simulink model "MyobsvIntegralSimul"  (R2021b)
settings: Solver=VariableStepAuto  StartTime=0.0  StopTime=200  RelTol=1e-3
undefined symbols (not defined in the file): A, B, C, F, G, Kd, Ki, L, Ts, x0, x_esht_0
settings Model: Creator=tanzc  LastModifiedBy=tanzc
settings DataIOCC: ReturnWorkspaceOutputs=off

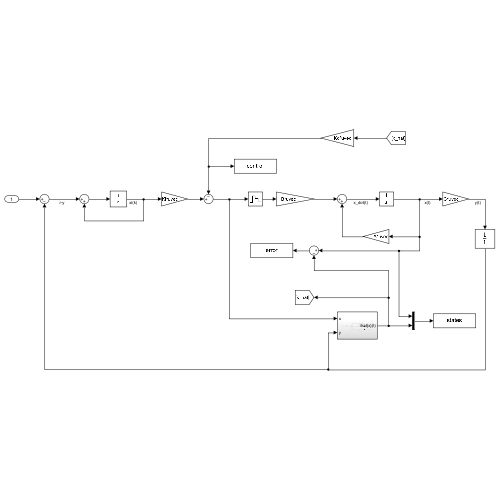
[thumbnail: Simulink's stored preview of the top-level diagram]
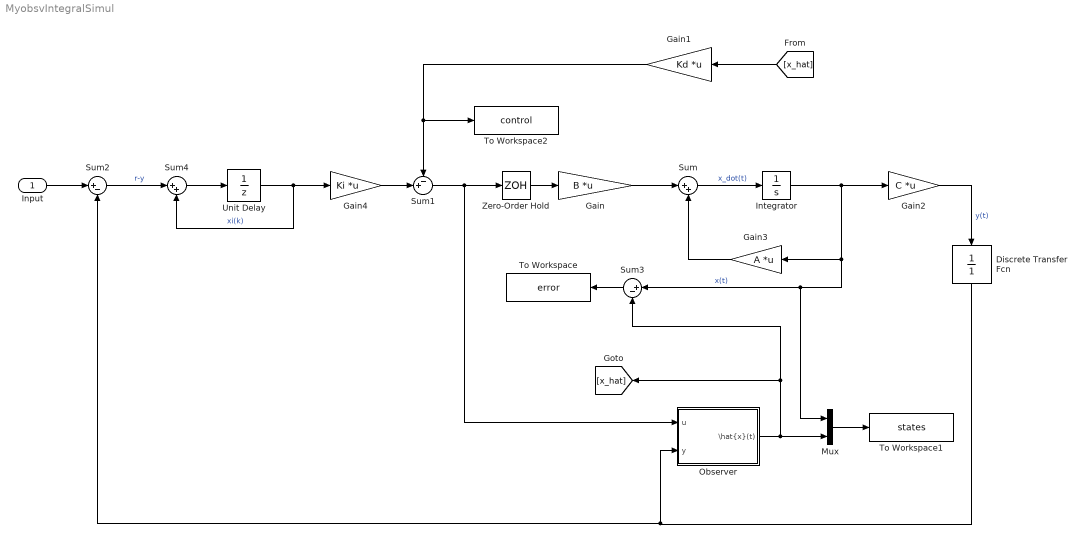
== system MyobsvIntegralSimul ==
  Input : Inport  PortDimensions=2
  Discrete Transfer Fcn : DiscreteTransferFcn  Denominator=1  SampleTime=Ts
  Gain : Gain  Gain=B  Multiplication=Matrix(K*u) (u vector)
  Gain1 : Gain  Gain=Kd  Multiplication=Matrix(K*u) (u vector)
  Gain2 : Gain  Gain=C  Multiplication=Matrix(K*u) (u vector)
  Gain3 : Gain  Gain=A  Multiplication=Matrix(K*u) (u vector)
  Gain4 : Gain  Gain=Ki  Multiplication=Matrix(K*u) (u vector)
  Integrator : Integrator  InitialCondition=x0
  Mux : Mux  Inputs=2
  Observer : Subsystem
  Sum : Sum  Inputs=|++
  Sum1 : Sum  Inputs=-+|
  Sum2 : Sum  Inputs=|+-
  Sum3 : Sum  Inputs=|+-
  Sum4 : Sum  Inputs=|++
  To Workspace : ToWorkspace  VariableName=error  SaveFormat=Structure With Time  SampleTime=-1
  To Workspace1 : ToWorkspace  VariableName=states  SaveFormat=Structure With Time  SampleTime=-1
  To Workspace2 : ToWorkspace  VariableName=control  SaveFormat=Structure With Time  SampleTime=-1
  Unit Delay : UnitDelay  SampleTime=Ts  HasFrameUpgradeWarning=on
  Zero-Order Hold : ZeroOrderHold  SampleTime=Ts
  wires:
  Gain/1 -> Sum/1
  Integrator/1 -> Mux/1, Sum3/1, Gain3/1, Gain2/1  "x(t)"
  Sum/1 -> Integrator/1  "x_dot(t)"
  Gain3/1 -> Sum/2
  Gain2/1 -> Discrete Transfer Fcn/1  "y(t)"
  Sum3/1 -> To Workspace/1
  Discrete Transfer Fcn/1 -> Sum2/2, Observer/2(y)
  Observer/1("\\hat{x}(t)") -> Mux/2, [x_hat], Sum3/2
  Mux/1 -> To Workspace1/1
  Gain1/1 -> To Workspace2/1, Sum1/1
  [x_hat] -> Gain1/1
  Sum1/1 -> Zero-Order Hold/1, Observer/1(u)
  Input/1 -> Sum2/1
  Sum4/1 -> Unit Delay/1
  Unit Delay/1 -> Gain4/1, Sum4/2  "xi(k)"
  Sum2/1 -> Sum4/1  "r-y"
  Gain4/1 -> Sum1/2
  Zero-Order Hold/1 -> Gain/1

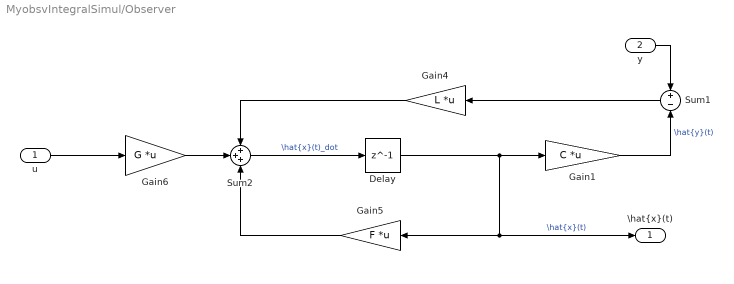
== system MyobsvIntegralSimul/Observer ==
  u : Inport
  y : Inport  Port=2
  Delay : Delay  DelayLength=1  InitialCondition=x_esht_0  SampleTime=Ts
  Gain1 : Gain  Gain=C  Multiplication=Matrix(K*u) (u vector)
  Gain4 : Gain  Gain=L  Multiplication=Matrix(K*u) (u vector)
  Gain5 : Gain  Gain=F  Multiplication=Matrix(K*u) (u vector)
  Gain6 : Gain  Gain=G  Multiplication=Matrix(K*u) (u vector)
  Sum1 : Sum  Inputs=+-
  Sum2 : Sum  Inputs=+++
  "\\hat{x}(t)" : Outport
  wires:
  y/1 -> Sum1/1
  Gain6/1 -> Sum2/2
  u/1 -> Gain6/1
  Gain4/1 -> Sum2/1
  Sum1/1 -> Gain4/1
  Delay/1 -> "\\hat{x}(t)"/1, Gain5/1, Gain1/1  "\\hat{x}(t)"
  Sum2/1 -> Delay/1  "\\hat{x}(t)_dot"
  Gain1/1 -> Sum1/2  "\\hat{y}(t)"
  Gain5/1 -> Sum2/3
